simulink model "VS_1_FPNSC_Ilimit_ok"  (R2013a)
settings: Solver=ode23tb  StartTime=0.0  StopTime=.65  RelTol=1e-3
PreLoadFcn:
  | t1=1;
InitFcn:
  | t_Pref1=0.07; Pref1=10e5;
  | t_Pref2=0.3;   Pref2=3e5;
  | 
  | t_Qmax1=.12; t_Qmax2=t_Qmax1+.01;
  | t_Qref1=0.09; Qref1=7e5;
  | t_Qref2=0.5; Qref2=10e5;
  | 
  | t_Imax1=.2; Imax1=1200;
  | t_Imax2=.4; Imax2=1500;
  | 
  | t_k1=0.25; k1=.8;
  | t_k2=0.35; k2=.2;
  | t_h1=0.45; h1=.9;
  | t_h2=0.55; h2=.5;
  | 
  | Lg=90e-6;
  | l=100e-6; r=2e-3;
  | tff=10e-6;
  | w=2*pi*60;
  | z_lead =966.3602;
  | p_lead =5.6324e+03;
  | Vdc=10000;
  | Vs=690;
undefined symbols (not defined in the file): magnitude
libraries: powerlib x39, powerlib_meascontrol x17, simulink x8, simulink_extras x3
settings Model: Creator=Shahed Mortazavian  LastModifiedBy=Shahed Mortazavian
settings DataIOCC: SignalLoggingSaveFormat=ModelDataLogs
settings OptimizationCC: ExpressionDepthLimit=2147483647
settings DebuggingCC: FcnCallInpInsideContextMsg=UseLocalSettings
settings GRTTargetCC: CombineOutputUpdateFcns=off  GRTInterface=on

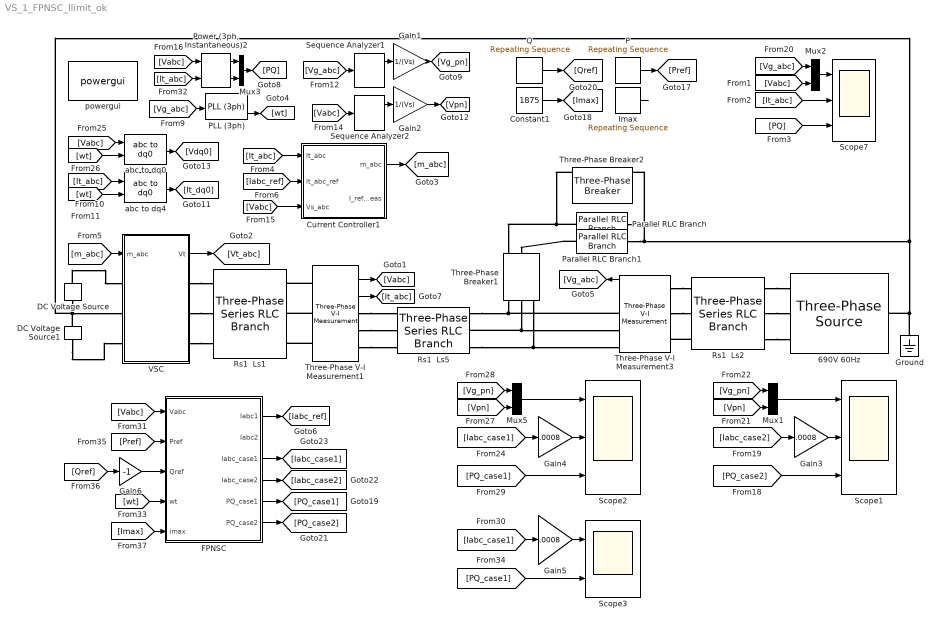
== system VS_1_FPNSC_Ilimit_ok ==
  690V 60Hz : powerlib/Electrical Sources/Three-Phase Source  Voltage=Vs*sqrt(3)/sqrt(2)  PhaseAngle=0  Frequency=60  InternalConnection=Yn  SpecifyImpedance=off  Resistance=2e-10  Inductance=1e-10  ShortCircuitLevel=100e6  BaseVoltage=25e3  XRratio=7  BusType=swing  Pref=0  Qref=0  Qmin=-inf  Qmax=inf
  Constant1 : Constant  Value=1875
  Current Controller1 : Subsystem
  DC Voltage Source : powerlib/Electrical Sources/DC Voltage Source  Amplitude=Vdc/2  Measurements=None
  DC Voltage Source1 : powerlib/Electrical Sources/DC Voltage Source  Amplitude=Vdc/2  Measurements=None
  FPNSC : Subsystem
  Gain1 : Gain  Gain=1/(Vs)
  Gain2 : Gain  Gain=1/(Vs)
  Gain3 : Gain  Gain=.0008
  Gain4 : Gain  Gain=.0008
  Gain5 : Gain  Gain=.0008
  Gain6 : Gain  Gain=-1
  Ground : powerlib/Elements/Ground  LConnTagsString=a
  Imax : simulink/Sources/Repeating Sequence  rep_seq_t=[0 t_Imax1 t_Imax1 t_Imax2 t_Imax2 10]  rep_seq_y=[1000 1000 Imax1 Imax1 Imax2 Imax2]
  Mux{1..3,5} (4 alike) : Mux  Inputs=2
  P : simulink/Sources/Repeating Sequence  rep_seq_t=[0 t_Pref1 t_Pref1 t_Pref2 t_Pref2 10]  rep_seq_y=2/3*[0 0 Pref1 Pref1 Pref2 Pref2]
  PLL (3ph) : powerlib_meascontrol/PLL/PLL (3ph)  Fmin=45  Par_Init=[0, 60]  ParK=[180, 3200, 1]  TcD=1e-4  MaxRateChangeFreq=12  FilterCutOffFreq=25  Ts=0  AGC=on
  Parallel RLC Branch : powerlib/Elements/Parallel RLC Branch  LConnTagsString=a  RConnTagsString=__new0  BranchType=R  Resistance=.8e-3  Inductance=1e-3  SetiL0=off  InitialCurrent=0  Capacitance=1e-6  Setx0=off  InitialVoltage=0  Measurements=None
  Parallel RLC Branch1 : powerlib/Elements/Parallel RLC Branch  LConnTagsString=a  RConnTagsString=__new0  BranchType=R  Resistance=.02  Inductance=1e-3  SetiL0=off  InitialCurrent=0  Capacitance=1e-6  Setx0=off  InitialVoltage=0  Measurements=None
  "Power (3ph, Instantaneous)2" : powerlib_meascontrol/Measurements/Power (3ph, Instantaneous)
  Q : simulink/Sources/Repeating Sequence  rep_seq_t=[0 t_Qref1 t_Qref1 t_Qref2 t_Qref2 10]  rep_seq_y=-2/3*[0 0 Qref1 Qref1 Qref2 Qref2]
  Rs1  Ls1 : powerlib/Elements/Three-Phase Series RLC Branch  LConnTagsString=A|B|C  RConnTagsString=A|B|C  BranchType=RL  Resistance=r  Inductance=l  Capacitance=1e-6  Measurements=None
  Rs1  Ls2 : powerlib/Elements/Three-Phase Series RLC Branch  LConnTagsString=A|B|C  RConnTagsString=A|B|C  BranchType=R  Resistance=1e-3  Inductance=l  Capacitance=1e-6  Measurements=None
  Rs1  Ls5 : powerlib/Elements/Three-Phase Series RLC Branch  LConnTagsString=A|B|C  RConnTagsString=A|B|C  BranchType=RL  Resistance=7e-3  Inductance=Lg  Capacitance=1e-6  Measurements=None
  Scope1 : Scope  NumInputPorts=3
      settings: YMin=2.77556e-17~-1~-1  YMax=1.1~1~1  SaveName=Data  Decimation=100  SampleInput=on
  Scope2 : Scope  NumInputPorts=3
      settings: YMin=2.77556e-17~-1~-500000  YMax=1.05~1~2.75e+06  SaveName=data_case1  Decimation=100  SampleInput=on
  Scope3 : Scope  NumInputPorts=2
      settings: YMin=-2~-1.5e+06  YMax=2~5.5e+06  SaveName=Data2  Decimation=100  SampleInput=on
  Scope7 : Scope  NumInputPorts=3
      settings: YMin=-1500~-1250~-1e+06  YMax=2000~1750~3e+06  SaveName=ScopeData9  Decimation=100  SampleInput=on
  Sequence Analyzer1 : powerlib_meascontrol/Measurements/Sequence Analyzer  Freq=60  n=1  seq=Positive Negative Zero  InInit=[1, 0]  Ts=0
  Sequence Analyzer2 : powerlib_meascontrol/Measurements/Sequence Analyzer  Freq=60  n=1  seq=Positive Negative Zero  InInit=[1, 0]  Ts=0
  Three-Phase V-I Measurement1 : powerlib/Measurements/Three-Phase V-I Measurement  VoltageMeasurement=phase-to-ground  SetLabelV=off  LabelV=Vabc  Vpu=off  VpuLL=off  CurrentMeasurement=yes  SetLabelI=off  LabelI=Iabc  Ipu=off  Pbase=100e6  Vbase=500e3  OutputType=Complex  PhasorSimulation=off  PSBequivalent=0
  Three-Phase V-I Measurement3 : powerlib/Measurements/Three-Phase V-I Measurement  VoltageMeasurement=phase-to-ground  SetLabelV=off  LabelV=Vabc  Vpu=off  VpuLL=off  CurrentMeasurement=yes  SetLabelI=off  LabelI=Iabc  Ipu=off  Pbase=100e6  Vbase=500e3  OutputType=Complex  PhasorSimulation=off  PSBequivalent=0
  Three-Phase Breaker1 : powerlib/Elements/Three-Phase Breaker  InitialState=open  SwitchA=on  SwitchB=on  SwitchC=on  SwitchTimes=[.2 10]  External=off  BreakerResistance=1e-40  SnubberResistance=1e6  SnubberCapacitance=inf  Measurements=None
  Three-Phase Breaker2 : powerlib/Elements/Three-Phase Breaker  InitialState=open  SwitchA=on  SwitchB=on  SwitchC=on  SwitchTimes=.4  External=off  BreakerResistance=1e-40  SnubberResistance=1e6  SnubberCapacitance=inf  Measurements=None
  VSC : Subsystem
  abc to dq0 : powerlib_meascontrol/Transformations/abc to dq0  Alignment=90 degrees behind phase A axis
  abc to dq4 : powerlib_meascontrol/Transformations/abc to dq0  Alignment=90 degrees behind phase A axis
  powergui : powerlib/powergui  Priority=2  SimulationMode=Discrete  SolverType=Tustin  SampleTime=5e-5  frequency=60  SPID=off  DisableSnubberDevices=off  DisableRonSwitches=off  DisableVfSwitches=off  SwTol=0  Interpol=off  DisplayEquations=off  frequencyindice=0  Pbase=100e6  ErrMax=1e-4  Iterations=50  UnitsV=kV  UnitsW=MW  FunctionMessages=off  echomessages=off  HookPort=off  EnableUseOfTLC=off  x0status=blocks  RestoreLinks=warning  ResistiveCurrentMeasurement=off  Frange=[0:2:500]  Ylog=off  Xlog=on  ShowGrid=off  save=off  variable=ZData  structure=Data  ZoomFFT=off  StartTime=.22  cycles=2  DisplayStyle=1  fundamental=60  FreqAxis=off  MaxFrequency=1000  frequencyindicesteady=1  RmsSteady=1  display=off  Ts=0  methode=off
  wires:
  "Power (3ph, Instantaneous)2"/1 -> Mux3/1
  "Power (3ph, Instantaneous)2"/2 -> Mux3/2
  Mux3/1 -> [PQ]
  [It_abc] -> Scope7/2
  [PQ] -> Scope7/3
  [Vg_abc] -> Sequence Analyzer1/1
  Sequence Analyzer1/1 -> Gain1/1
  Gain1/1 -> [Vg_pn]
  Three-Phase V-I Measurement1/1 -> [Vabc]
  VSC/1(Vt) -> [Vt_abc]
  [m_abc] -> VSC/1(m_abc)
  Three-Phase V-I Measurement3/1 -> [Vg_abc]
  [Vabc] -> abc to dq0/1
  [wt] -> abc to dq0/2
  abc to dq0/1 -> [Vdq0]
  [It_abc] -> abc to dq4/1
  abc to dq4/1 -> [It_dq0]
  [wt] -> abc to dq4/2
  [Vg_abc] -> PLL (3ph)/1
  [Vabc] -> "Power (3ph, Instantaneous)2"/1
  [It_abc] -> "Power (3ph, Instantaneous)2"/2
  PLL (3ph)/2 -> [wt]
  P/1 -> [Pref]
  Imax/1 -> ?
  Q/1 -> [Qref]
  Constant1/1 -> [Imax]
  [Vpn] -> Mux1/2
  [Vg_pn] -> Mux1/1
  [PQ_case2] -> Scope1/3
  Gain3/1 -> Scope1/2
  Mux1/1 -> Scope1/1
  Three-Phase V-I Measurement1/2 -> [It_abc]
  Mux2/1 -> Scope7/1
  [Vabc] -> Mux2/2
  [Vg_abc] -> Mux2/1
  [Vabc] -> Sequence Analyzer2/1
  Sequence Analyzer2/1 -> Gain2/1
  Gain2/1 -> [Vpn]
  [Iabc_case2] -> Gain3/1
  [Vpn] -> Mux5/2
  [Vg_pn] -> Mux5/1
  Mux5/1 -> Scope2/1
  Gain4/1 -> Scope2/2
  [Iabc_case1] -> Gain4/1
  [PQ_case1] -> Scope2/3
  Gain5/1 -> Scope3/1
  [Iabc_case1] -> Gain5/1
  [PQ_case1] -> Scope3/2
  [wt] -> FPNSC/4(wt)
  [Vabc] -> FPNSC/1(Vabc)
  [Pref] -> FPNSC/2(Pref)
  [Qref] -> Gain6/1
  [Imax] -> FPNSC/5(imax)
  FPNSC/3(Iabc_case1) -> [Iabc_case1]
  FPNSC/4(Iabc_case2) -> [Iabc_case2]
  FPNSC/5(PQ_case1) -> [PQ_case1]
  FPNSC/6(PQ_case2) -> [PQ_case2]
  [It_abc] -> Current Controller1/1(It_abc)
  [Vabc] -> Current Controller1/3(Vs_abc)
  Current Controller1/1(m_abc) -> [m_abc]
  FPNSC/1(Iabc1) -> [Iabc_ref]
  [Iabc_ref] -> Current Controller1/2(It_abc_ref)
  Gain6/1 -> FPNSC/3(Qref)
  connections:
  Three-Phase V-I Measurement1/LConn1 -- Rs1  Ls1/RConn1
  Three-Phase V-I Measurement1/LConn2 -- Rs1  Ls1/RConn2
  Three-Phase V-I Measurement1/LConn3 -- Rs1  Ls1/RConn3
  Rs1  Ls5/RConn1 -- Three-Phase V-I Measurement3/RConn1 -- Three-Phase Breaker1/LConn1
  Three-Phase Breaker2/LConn1 -- Parallel RLC Branch/LConn1 -- Three-Phase Breaker1/RConn1
  VSC/RConn1 -- Rs1  Ls1/LConn1
  VSC/RConn2 -- Rs1  Ls1/LConn2
  VSC/RConn3 -- Rs1  Ls1/LConn3
  DC Voltage Source/RConn1 -- VSC/LConn1
  DC Voltage Source1/LConn1 -- VSC/LConn3
  Three-Phase Breaker1/LConn2 -- Rs1  Ls5/RConn2 -- Three-Phase V-I Measurement3/RConn2
  Rs1  Ls5/RConn3 -- Three-Phase Breaker1/LConn3 -- Three-Phase V-I Measurement3/RConn3
  Three-Phase V-I Measurement3/LConn1 -- Rs1  Ls2/LConn1
  Three-Phase V-I Measurement3/LConn2 -- Rs1  Ls2/LConn2
  Rs1  Ls2/LConn3 -- Three-Phase V-I Measurement3/LConn3
  Rs1  Ls2/RConn1 -- 690V 60Hz/RConn1
  Rs1  Ls2/RConn2 -- 690V 60Hz/RConn2
  Rs1  Ls2/RConn3 -- 690V 60Hz/RConn3
  Parallel RLC Branch1/LConn1 -- Three-Phase Breaker1/RConn2
  Three-Phase V-I Measurement1/RConn1 -- Rs1  Ls5/LConn1
  Three-Phase V-I Measurement1/RConn2 -- Rs1  Ls5/LConn2
  Three-Phase V-I Measurement1/RConn3 -- Rs1  Ls5/LConn3
  DC Voltage Source/LConn1 -- DC Voltage Source1/RConn1 -- Parallel RLC Branch1/RConn1 -- Three-Phase Breaker2/RConn1 -- Parallel RLC Branch/RConn1 -- Ground/LConn1 -- 690V 60Hz/LConn1 -- VSC/LConn2

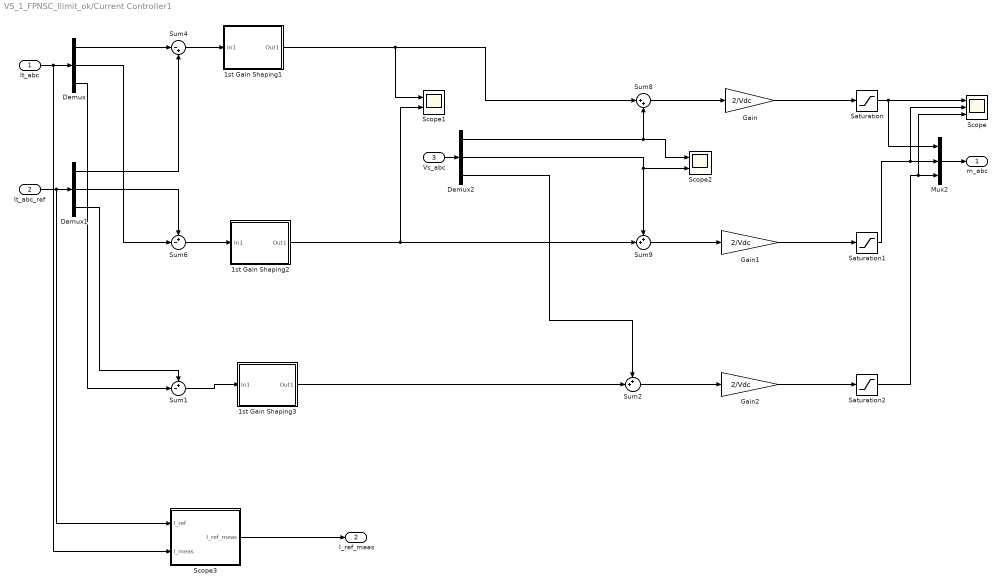
== system VS_1_FPNSC_Ilimit_ok/Current Controller1 ==
  It_abc : Inport
  It_abc_ref : Inport  Port=2
  Vs_abc : Inport  Port=3
  1st Gain Shaping1 : Subsystem
  1st Gain Shaping2 : Subsystem
  1st Gain Shaping3 : Subsystem
  Demux : Demux  Outputs=3
  Demux1 : Demux  Outputs=3
  Demux2 : Demux  Outputs=3
  Gain : Gain  Gain=2/Vdc
  Gain1 : Gain  Gain=2/Vdc
  Gain2 : Gain  Gain=2/Vdc
  Mux2 : Mux  Inputs=3
  Saturation : Saturate  UpperLimit=1  LowerLimit=-1
  Saturation1 : Saturate  UpperLimit=1  LowerLimit=-1
  Saturation2 : Saturate  UpperLimit=1  LowerLimit=-1
  Scope : Scope  NumInputPorts=3
      settings: YMin=-0.7~-1~-0.75  YMax=0.8~0.75~1  SaveName=ScopeData4  Decimation=3
  Scope1 : Scope  NumInputPorts=2
      settings: YMin=-1600~-200  YMax=400~600  SaveName=ScopeData3  Decimation=3
  Scope2 : Scope  NumInputPorts=2
      settings: YMin=-400~-450  YMax=400~400  SaveName=ScopeData5  Decimation=3
  Scope3 : Subsystem
  Sum1 : Sum  Inputs=+-|
  Sum2 : Sum  Inputs=++|
  Sum4 : Sum  Inputs=|-+
  Sum6 : Sum  Inputs=+-|
  Sum8 : Sum  Inputs=|++
  Sum9 : Sum  Inputs=++|
  m_abc : Outport
  I_ref_meas : Outport  Port=2
  wires:
  Demux2/1 -> Scope2/1, Sum8/2
  Demux2/2 -> Scope2/2, Sum9/1
  Sum6/1 -> 1st Gain Shaping2/1(In1)
  It_abc/1 -> Scope3/2(I_meas), Demux/1
  It_abc_ref/1 -> Scope3/1(I_ref), Demux1/1
  Vs_abc/1 -> Demux2/1
  Sum8/1 -> Gain/1
  Sum9/1 -> Gain1/1
  Mux2/1 -> m_abc/1
  Gain/1 -> Saturation/1
  Gain1/1 -> Saturation1/1
  Saturation2/1 -> Scope/3, Mux2/3
  Saturation/1 -> Scope/1, Mux2/1
  Saturation1/1 -> Mux2/2, Scope/2
  Demux1/1 -> Sum4/2
  Demux/1 -> Sum4/1
  Sum4/1 -> 1st Gain Shaping1/1(In1)
  Demux1/2 -> Sum6/1
  Demux/2 -> Sum6/2
  Demux1/3 -> Sum1/1
  Demux/3 -> Sum1/2
  Sum1/1 -> 1st Gain Shaping3/1(In1)
  Gain2/1 -> Saturation2/1
  Sum2/1 -> Gain2/1
  Demux2/3 -> Sum2/1
  1st Gain Shaping2/1(Out1) -> Scope1/2, Sum9/2
  1st Gain Shaping3/1(Out1) -> Sum2/2
  1st Gain Shaping1/1(Out1) -> Scope1/1, Sum8/1
  Scope3/1(I_ref_meas) -> I_ref_meas/1

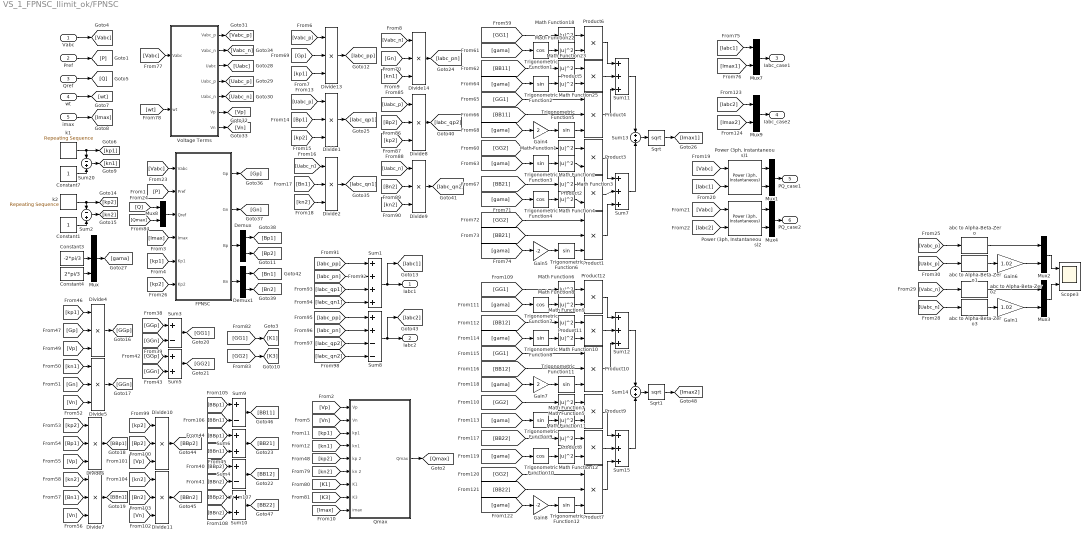
== system VS_1_FPNSC_Ilimit_ok/FPNSC ==
  Vabc : Inport
  Pref : Inport  Port=2
  Qref : Inport  Port=3
  wt : Inport  Port=4
  imax : Inport  Port=5
  Constant1 : Constant
  Constant3 : Constant  Value=-2*pi/3
  Constant4 : Constant  Value=2*pi/3
  Constant7 : Constant
  Demux : Demux  Outputs=2
  Demux1 : Demux  Outputs=2
  Divide{1..2,4..11,13..14} (12 alike) : Product  Inputs=***
  FPNSC : Subsystem
  Gain1 : Gain  Gain=1.02
  Gain4 : Gain  Gain=2
  Gain5 : Gain  Gain=-2
  Gain6 : Gain  Gain=1.02
  Gain7 : Gain  Gain=2
  Gain8 : Gain  Gain=-2
  Math Function{1..12,18,22..23,25} (16 alike) : Math  Operator=magnitude^2  SaturateOnIntegerOverflow=on
  Mux : Mux  Inputs=3
  Mux{1..4,7..9} (7 alike) : Mux  Inputs=2
  "Power (3ph, Instantaneous)1" : powerlib_meascontrol/Measurements/Power (3ph, Instantaneous)
  "Power (3ph, Instantaneous)2" : powerlib_meascontrol/Measurements/Power (3ph, Instantaneous)
  Product{1,4,7,10} (4 alike) : Product  Inputs=3
  Product{2..3,5..6,8..9,11..12} (8 alike) : Product
  Qmax : Subsystem
  Scope3 : Scope  NumInputPorts=2
      settings: YMin=-800~-70  YMax=800~70  SaveName=ScopeData11
  Sqrt : Sqrt  SaturateOnIntegerOverflow=on
  Sqrt1 : Sqrt  SaturateOnIntegerOverflow=on
  Sum1 : Sum  Inputs=++++
  Sum{5..6,10,13..14} (5 alike) : Sum
  Sum{7,11..12,15} (4 alike) : Sum  Inputs=+++
  Sum2 : Sum  Inputs=-+
  Sum20 : Sum  Inputs=-+
  Sum3 : Sum  Inputs=+-
  Sum4 : Sum  Inputs=+-
  Sum8 : Sum  Inputs=++--
  Sum9 : Sum  Inputs=+-
  Trigonometric Function{1,4,7,10} (4 alike) : Trigonometry  Operator=cos
  Trigonometric Function{2..3,5..6,8..9,11..12} (8 alike) : Trigonometry
  Voltage Terms : Subsystem
  abc to Alpha-Beta-Zero{,1..3} (4 alike) : powerlib_meascontrol/Transformations/abc to Alpha-Beta-Zero
  k1 : simulink/Sources/Repeating Sequence  rep_seq_t=[0 t_k1 t_k1 t_k2 t_k2 10]  rep_seq_y=[1 1 k1 k1 k2 k2]
  k2 : simulink/Sources/Repeating Sequence  rep_seq_t=[0 t_h1 t_h1 t_h2 t_h2 10]  rep_seq_y=[1 1 h1 h1 h2 h2]
  Iabc1 : Outport
  Iabc2 : Outport  Port=2
  Iabc_case1 : Outport  Port=3
  Iabc_case2 : Outport  Port=4
  PQ_case1 : Outport  Port=5
  PQ_case2 : Outport  Port=6
  wires:
  Divide13/1 -> [Iabc_pp]
  [kp1] -> FPNSC/5(Kp1)
  [Imax] -> FPNSC/4(Imax)
  [P] -> FPNSC/2(Pref)
  [Vabc] -> FPNSC/1(Vabc)
  Mux1/1 -> PQ_case1/1
  "Power (3ph, Instantaneous)1"/2 -> Mux1/2
  "Power (3ph, Instantaneous)1"/1 -> Mux1/1
  [Iabc1] -> "Power (3ph, Instantaneous)1"/2
  [Vabc] -> "Power (3ph, Instantaneous)1"/1
  Sum1/1 -> Iabc1/1, [Iabc1]
  [kn2] -> Divide2/3
  [Bn1] -> Divide2/2
  [Uabc_n] -> Divide2/1
  [kp2] -> Divide1/3
  [Uabc_p] -> Divide1/1
  [kn1] -> Divide14/3
  [Vabc_n] -> Divide14/1
  [kp1] -> Divide13/3
  Sum20/1 -> [kn1]
  k1/1 -> [kp1], Sum20/1
  [Vabc_p] -> Divide13/1
  imax/1 -> [Imax]
  wt/1 -> [wt]
  Qref/1 -> [Q]
  Pref/1 -> [P]
  Vabc/1 -> [Vabc]
  FPNSC/4(Bn) -> Demux1/1
  FPNSC/2(Gn) -> [Gn]
  Constant7/1 -> Sum20/2
  [Gp] -> Divide13/2
  [Gn] -> Divide14/2
  [Vabc_p] -> abc to Alpha-Beta-Zero/1
  [Uabc_p] -> abc to Alpha-Beta-Zero1/1
  [Vabc_n] -> abc to Alpha-Beta-Zero2/1
  [Uabc_n] -> abc to Alpha-Beta-Zero3/1
  abc to Alpha-Beta-Zero/1 -> Mux2/1
  abc to Alpha-Beta-Zero1/1 -> Gain6/1
  abc to Alpha-Beta-Zero2/1 -> Mux3/1
  abc to Alpha-Beta-Zero3/1 -> Gain1/1
  Mux2/1 -> Scope3/1
  Mux3/1 -> Scope3/2
  Gain6/1 -> Mux2/2
  Gain1/1 -> Mux3/2
  Sum2/1 -> [kn2]
  k2/1 -> Sum2/1, [kp2]
  Constant1/1 -> Sum2/2
  [kp2] -> FPNSC/6(Kp2)
  [GGp] -> Sum3/1
  [GGn] -> Sum3/2
  Sum3/1 -> [GG1]
  [BBp2] -> Sum4/1
  [BBn2] -> Sum4/2
  Sum4/1 -> [BB12]
  [GGp] -> Sum5/1
  [GGn] -> Sum5/2
  Sum5/1 -> [GG2]
  [BBp1] -> Sum6/1
  [BBn1] -> Sum6/2
  Sum6/1 -> [BB21]
  [kp1] -> Divide4/1
  [Gp] -> Divide4/2
  [Vp] -> Divide4/3
  Divide4/1 -> [GGp]
  [kn1] -> Divide5/1
  [Gn] -> Divide5/2
  [Vn] -> Divide5/3
  Divide5/1 -> [GGn]
  Divide6/1 -> [BBp1]
  Divide7/1 -> [BBn1]
  [kp2] -> Divide6/1
  [Bp1] -> Divide6/2
  [Vp] -> Divide6/3
  [Vn] -> Divide7/3
  [Bn1] -> Divide7/2
  [kn2] -> Divide7/1
  [GG1] -> Math Function18/1
  [gama] -> Trigonometric Function1/1
  Trigonometric Function1/1 -> Math Function22/1
  Math Function22/1 -> Product6/2
  Math Function18/1 -> Product6/1
  Math Function23/1 -> Product5/1
  Math Function25/1 -> Product5/2
  [BB11] -> Math Function23/1
  [gama] -> Trigonometric Function2/1
  Trigonometric Function2/1 -> Math Function25/1
  [GG1] -> Product4/1
  [BB11] -> Product4/2
  [gama] -> Gain4/1
  Product6/1 -> Sum11/1
  Product5/1 -> Sum11/2
  Product4/1 -> Sum11/3
  Sum11/1 -> Sum13/1
  Sum7/1 -> Sum13/2
  Sum13/1 -> Sqrt/1
  Gain4/1 -> Trigonometric Function5/1
  Trigonometric Function5/1 -> Product4/3
  [GG2] -> Math Function1/1
  [gama] -> Trigonometric Function3/1
  Trigonometric Function3/1 -> Math Function2/1
  Math Function2/1 -> Product3/2
  Math Function1/1 -> Product3/1
  Math Function3/1 -> Product2/1
  Math Function4/1 -> Product2/2
  [BB21] -> Math Function3/1
  [gama] -> Trigonometric Function4/1
  Trigonometric Function4/1 -> Math Function4/1
  [GG2] -> Product1/1
  [BB21] -> Product1/2
  [gama] -> Gain5/1
  Product3/1 -> Sum7/1
  Product2/1 -> Sum7/2
  Product1/1 -> Sum7/3
  Gain5/1 -> Trigonometric Function6/1
  Trigonometric Function6/1 -> Product1/3
  [Iabc1] -> Mux7/1
  Sqrt/1 -> [Imax1]
  [Imax1] -> Mux7/2
  Mux7/1 -> Iabc_case1/1
  Constant3/1 -> Mux/2
  Constant4/1 -> Mux/3
  Mux/1 -> [gama]
  [wt] -> Voltage Terms/2(wt)
  [Vabc] -> Voltage Terms/1(Vabc)
  Voltage Terms/1(Vabc_p) -> [Vabc_p]
  Voltage Terms/2(Vabc_n) -> [Vabc_n]
  Voltage Terms/3(Uabc) -> [Uabc]
  Voltage Terms/4(Uabc_p) -> [Uabc_p]
  Voltage Terms/5(Uabc_n) -> [Uabc_n]
  Voltage Terms/6(Vp) -> [Vp]
  Voltage Terms/7(Vn) -> [Vn]
  [Vn] -> Qmax/2(Vn)
  [kp1] -> Qmax/3(kp1)
  [Vp] -> Qmax/1(Vp)
  [Imax] -> Qmax/9(imax)
  Qmax/1(Qmax) -> [Qmax]
  [kn1] -> Qmax/4(kn1)
  [kp2] -> Qmax/5(kp 2)
  [kn2] -> Qmax/6(kn 2)
  [K1] -> Qmax/7(K1)
  [K3] -> Qmax/8(K3)
  [GG1] -> [K1]
  [GG2] -> [K3]
  [Q] -> Mux8/1
  [Qmax] -> Mux8/2
  Mux8/1 -> FPNSC/3(Qref)
  FPNSC/1(Gp) -> [Gp]
  FPNSC/3(Bp) -> Demux/1
  Demux/1 -> [Bp1]
  Demux/2 -> [Bp2]
  Divide14/1 -> [Iabc_pn]
  Divide1/1 -> [Iabc_qp1]
  [Bp1] -> Divide1/2
  Divide2/1 -> [Iabc_qn1]
  [kn2] -> Divide9/3
  [Bn2] -> Divide9/2
  [Uabc_n] -> Divide9/1
  [kp2] -> Divide8/3
  [Uabc_p] -> Divide8/1
  Divide8/1 -> [Iabc_qp2]
  [Bp2] -> Divide8/2
  Divide9/1 -> [Iabc_qn2]
  Demux1/1 -> [Bn1]
  Demux1/2 -> [Bn2]
  [Iabc_pp] -> Sum1/1
  [Iabc_pn] -> Sum1/2
  [Iabc_qp1] -> Sum1/3
  [Iabc_qn1] -> Sum1/4
  Sum8/1 -> Iabc2/1, [Iabc2]
  [Iabc_pp] -> Sum8/1
  [Iabc_pn] -> Sum8/2
  [Iabc_qp2] -> Sum8/3
  [Iabc_qn2] -> Sum8/4
  Divide10/1 -> [BBp2]
  Divide11/1 -> [BBn2]
  [kp2] -> Divide10/1
  [Bp2] -> Divide10/2
  [Vp] -> Divide10/3
  [Vn] -> Divide11/3
  [Bn2] -> Divide11/2
  [kn2] -> Divide11/1
  [BBp1] -> Sum9/1
  [BBn1] -> Sum9/2
  Sum9/1 -> [BB11]
  [BBp2] -> Sum10/1
  [BBn2] -> Sum10/2
  Sum10/1 -> [BB22]
  [GG1] -> Math Function6/1
  [gama] -> Trigonometric Function7/1
  Trigonometric Function7/1 -> Math Function8/1
  Math Function8/1 -> Product12/2
  Math Function6/1 -> Product12/1
  Math Function9/1 -> Product11/1
  Math Function10/1 -> Product11/2
  [BB12] -> Math Function9/1
  [gama] -> Trigonometric Function8/1
  Trigonometric Function8/1 -> Math Function10/1
  [GG1] -> Product10/1
  [BB12] -> Product10/2
  [gama] -> Gain7/1
  Product12/1 -> Sum12/1
  Product11/1 -> Sum12/2
  Product10/1 -> Sum12/3
  Sum12/1 -> Sum14/1
  Sum15/1 -> Sum14/2
  Sum14/1 -> Sqrt1/1
  Gain7/1 -> Trigonometric Function11/1
  Trigonometric Function11/1 -> Product10/3
  [GG2] -> Math Function5/1
  [gama] -> Trigonometric Function9/1
  Trigonometric Function9/1 -> Math Function7/1
  Math Function7/1 -> Product9/2
  Math Function5/1 -> Product9/1
  Math Function11/1 -> Product8/1
  Math Function12/1 -> Product8/2
  [BB22] -> Math Function11/1
  [gama] -> Trigonometric Function10/1
  Trigonometric Function10/1 -> Math Function12/1
  [GG2] -> Product7/1
  [BB22] -> Product7/2
  [gama] -> Gain8/1
  Product9/1 -> Sum15/1
  Product8/1 -> Sum15/2
  Product7/1 -> Sum15/3
  Gain8/1 -> Trigonometric Function12/1
  Trigonometric Function12/1 -> Product7/3
  Sqrt1/1 -> [Imax2]
  [Iabc2] -> Mux9/1
  [Imax2] -> Mux9/2
  Mux9/1 -> Iabc_case2/1
  Mux4/1 -> PQ_case2/1
  "Power (3ph, Instantaneous)2"/2 -> Mux4/2
  "Power (3ph, Instantaneous)2"/1 -> Mux4/1
  [Iabc2] -> "Power (3ph, Instantaneous)2"/2
  [Vabc] -> "Power (3ph, Instantaneous)2"/1

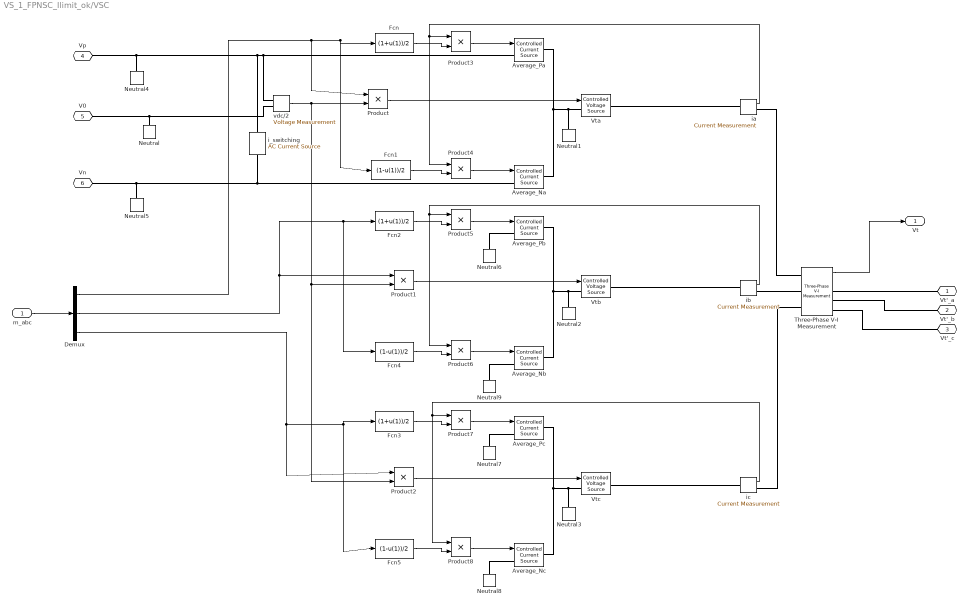
== system VS_1_FPNSC_Ilimit_ok/VSC ==
  m_abc : Inport
  Average_Na : powerlib/Electrical Sources/Controlled Current Source  Initialize=on  Source_Type=AC  Amplitude=0  Phase=0  Frequency=0  Measurements=None
  Average_Nb : powerlib/Electrical Sources/Controlled Current Source  Initialize=on  Source_Type=AC  Amplitude=0  Phase=0  Frequency=0  Measurements=None
  Average_Nc : powerlib/Electrical Sources/Controlled Current Source  Initialize=on  Source_Type=AC  Amplitude=0  Phase=0  Frequency=0  Measurements=None
  Average_Pa : powerlib/Electrical Sources/Controlled Current Source  Initialize=on  Source_Type=AC  Amplitude=0  Phase=0  Frequency=0  Measurements=None
  Average_Pb : powerlib/Electrical Sources/Controlled Current Source  Initialize=on  Source_Type=AC  Amplitude=0  Phase=0  Frequency=0  Measurements=None
  Average_Pc : powerlib/Electrical Sources/Controlled Current Source  Initialize=on  Source_Type=AC  Amplitude=0  Phase=0  Frequency=0  Measurements=None
  Demux : Demux  Outputs=3
  Fcn : Fcn  Expr=(1+u(1))/2
  Fcn1 : Fcn  Expr=(1-u(1))/2
  Fcn2 : Fcn  Expr=(1+u(1))/2
  Fcn3 : Fcn  Expr=(1+u(1))/2
  Fcn4 : Fcn  Expr=(1-u(1))/2
  Fcn5 : Fcn  Expr=(1-u(1))/2
  Neutral{,1..3} (4 alike) : powerlib/Elements/Neutral  LConnTagsString=a  NodeNumber=10
  Neutral4 : powerlib/Elements/Neutral  LConnTagsString=a  NodeNumber=11
  Neutral5 : powerlib/Elements/Neutral  LConnTagsString=a  NodeNumber=12
  Neutral6 : powerlib/Elements/Neutral  LConnTagsString=a  NodeNumber=11
  Neutral7 : powerlib/Elements/Neutral  LConnTagsString=a  NodeNumber=11
  Neutral8 : powerlib/Elements/Neutral  LConnTagsString=a  NodeNumber=12
  Neutral9 : powerlib/Elements/Neutral  LConnTagsString=a  NodeNumber=12
  Product{,1..8} (9 alike) : Product  RndMeth=Zero
  Three-Phase V-I Measurement : powerlib/Measurements/Three-Phase V-I Measurement  VoltageMeasurement=phase-to-ground  SetLabelV=off  LabelV=Vabc  Vpu=off  VpuLL=off  CurrentMeasurement=yes  SetLabelI=off  LabelI=Iabc  Ipu=off  Pbase=100e6  Vbase=500e3  OutputType=Complex  PhasorSimulation=off  PSBequivalent=0
  Vta : powerlib/Electrical Sources/Controlled Voltage Source  Initialize=on  Source_Type=AC  Amplitude=0  Phase=0  Frequency=0  Measurements=None
  Vtb : powerlib/Electrical Sources/Controlled Voltage Source  Initialize=on  Source_Type=AC  Amplitude=0  Phase=0  Frequency=0  Measurements=None
  Vtc : powerlib/Electrical Sources/Controlled Voltage Source  Initialize=on  Source_Type=AC  Amplitude=0  Phase=0  Frequency=0  Measurements=None
  i_switching : powerlib/Electrical Sources/AC Current Source  Amplitude=1  Phase=0  Frequency=0  SampleTime=0  Measurements=None
  ia : powerlib/Measurements/Current Measurement  PhasorSimulation=off  OutputType=Complex  PSBequivalent=0
  ib : powerlib/Measurements/Current Measurement  PhasorSimulation=off  OutputType=Complex  PSBequivalent=0
  ic : powerlib/Measurements/Current Measurement  PhasorSimulation=off  OutputType=Complex  PSBequivalent=0
  vdc/2 : powerlib/Measurements/Voltage Measurement  PhasorSimulation=off  OutputType=Complex  PSBequivalent=0
  Vt'_a : PMIOPort  Port=1  Side=Right
  Vt'_b : PMIOPort  Port=2  Side=Right
  Vt'_c : PMIOPort  Port=3  Side=Right
  Vp : PMIOPort  Port=4  Side=Left
  V0 : PMIOPort  Port=5  Side=Left
  Vn : PMIOPort  Port=6  Side=Left
  Vt : Outport
  wires:
  Fcn1/1 -> Product4/2
  Fcn2/1 -> Product5/2
  Fcn4/1 -> Product6/2
  Fcn3/1 -> Product7/2
  Fcn5/1 -> Product8/2
  Demux/1 -> Fcn/1, Fcn1/1, Product/1
  Demux/2 -> Fcn2/1, Fcn4/1, Product1/1
  Demux/3 -> Fcn3/1, Fcn5/1, Product2/1
  vdc/2/1 -> Product/2, Product1/2, Product2/2
  Product/1 -> Vta/1
  Product1/1 -> Vtb/1
  Product2/1 -> Vtc/1
  Product3/1 -> Average_Pa/1
  Fcn/1 -> Product3/2
  Product4/1 -> Average_Na/1
  Product5/1 -> Average_Pb/1
  Product7/1 -> Average_Pc/1
  Product8/1 -> Average_Nc/1
  ia/1 -> Product3/1, Product4/1
  ib/1 -> Product5/1, Product6/1
  ic/1 -> Product7/1, Product8/1
  Product6/1 -> Average_Nb/1
  m_abc/1 -> Demux/1
  Three-Phase V-I Measurement/1 -> Vt/1
  connections:
  Vn/RConn1 -- i_switching/RConn1 -- Average_Na/LConn1 -- Neutral5/LConn1
  Vp/RConn1 -- vdc/2/LConn1 -- Average_Pa/LConn1 -- i_switching/LConn1 -- Neutral4/LConn1
  Vta/RConn1 -- ia/LConn1
  Vtb/RConn1 -- ib/LConn1
  Vtc/RConn1 -- ic/LConn1
  Average_Pb/RConn1 -- Average_Nb/RConn1 -- Vtb/LConn1 -- Neutral2/LConn1
  Three-Phase V-I Measurement/LConn1 -- ia/RConn1
  Three-Phase V-I Measurement/LConn2 -- ib/RConn1
  Three-Phase V-I Measurement/LConn3 -- ic/RConn1
  Average_Pa/RConn1 -- Average_Na/RConn1 -- Vta/LConn1 -- Neutral1/LConn1
  Average_Pc/RConn1 -- Average_Nc/RConn1 -- Vtc/LConn1 -- Neutral3/LConn1
  V0/RConn1 -- vdc/2/LConn2 -- Neutral/LConn1
  Neutral6/LConn1 -- Average_Pb/LConn1
  Neutral7/LConn1 -- Average_Pc/LConn1
  Neutral8/LConn1 -- Average_Nc/LConn1
  Neutral9/LConn1 -- Average_Nb/LConn1
  Vt'_a/RConn1 -- Three-Phase V-I Measurement/RConn1
  Three-Phase V-I Measurement/RConn2 -- Vt'_b/RConn1
  Three-Phase V-I Measurement/RConn3 -- Vt'_c/RConn1

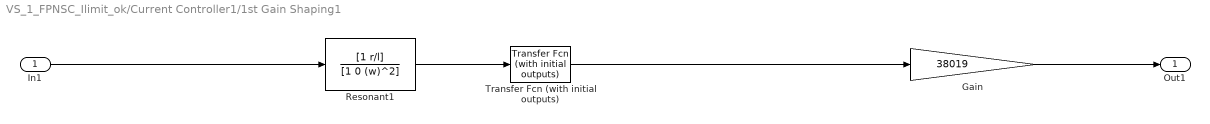
== system VS_1_FPNSC_Ilimit_ok/Current Controller1/1st Gain Shaping1 ==
  In1 : Inport
  Gain : Gain  Gain=38019
  Resonant1 : TransferFcn  Numerator=[1 r/l]  Denominator=[1 0 (w)^2]
  Transfer Fcn (with initial outputs) : simulink_extras/Additional Linear/Transfer Fcn (with initial outputs)  N=[1 5205]  D=[1 30340]  Y0=0  U0=0
  Out1 : Outport
  wires:
  Resonant1/1 -> Transfer Fcn (with initial outputs)/1
  In1/1 -> Resonant1/1
  Gain/1 -> Out1/1
  Transfer Fcn (with initial outputs)/1 -> Gain/1

== system VS_1_FPNSC_Ilimit_ok/Current Controller1/1st Gain Shaping2 ==
  In1 : Inport
  Gain : Gain  Gain=38019
  Resonant1 : TransferFcn  Numerator=[1 r/l]  Denominator=[1 0 (w)^2]
  Transfer Fcn (with initial outputs) : simulink_extras/Additional Linear/Transfer Fcn (with initial outputs)  N=[1 5205]  D=[1 30340]  Y0=0  U0=0
  Out1 : Outport
  wires:
  Transfer Fcn (with initial outputs)/1 -> Gain/1
  Gain/1 -> Out1/1
  In1/1 -> Resonant1/1
  Resonant1/1 -> Transfer Fcn (with initial outputs)/1

== system VS_1_FPNSC_Ilimit_ok/Current Controller1/1st Gain Shaping3 ==
  In1 : Inport
  Gain : Gain  Gain=38019
  Resonant1 : TransferFcn  Numerator=[1 r/l]  Denominator=[1 0 (w)^2]
  Transfer Fcn (with initial outputs) : simulink_extras/Additional Linear/Transfer Fcn (with initial outputs)  N=[1 5205]  D=[1 30340]  Y0=0  U0=0
  Out1 : Outport
  wires:
  Resonant1/1 -> Transfer Fcn (with initial outputs)/1
  In1/1 -> Resonant1/1
  Gain/1 -> Out1/1
  Transfer Fcn (with initial outputs)/1 -> Gain/1

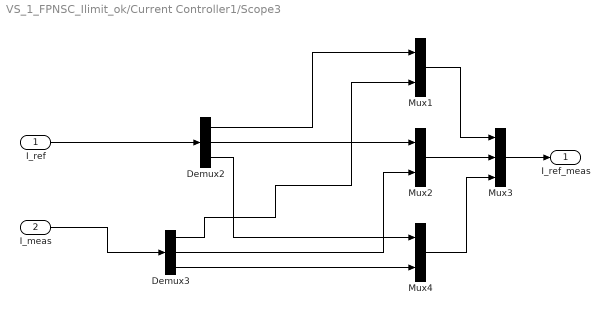
== system VS_1_FPNSC_Ilimit_ok/Current Controller1/Scope3 ==
  I_ref : Inport
  I_meas : Inport  Port=2
  Demux2 : Demux  Outputs=3
  Demux3 : Demux  Outputs=3
  Mux1 : Mux  Inputs=2
  Mux2 : Mux  Inputs=2
  Mux3 : Mux  Inputs=3
  Mux4 : Mux  Inputs=2
  I_ref_meas : Outport
  wires:
  I_meas/1 -> Demux3/1
  I_ref/1 -> Demux2/1
  Demux2/1 -> Mux1/1
  Demux3/1 -> Mux1/2
  Mux1/1 -> Mux3/1
  Demux2/2 -> Mux2/1
  Demux3/2 -> Mux2/2
  Mux2/1 -> Mux3/2
  Demux2/3 -> Mux4/1
  Demux3/3 -> Mux4/2
  Mux4/1 -> Mux3/3
  Mux3/1 -> I_ref_meas/1

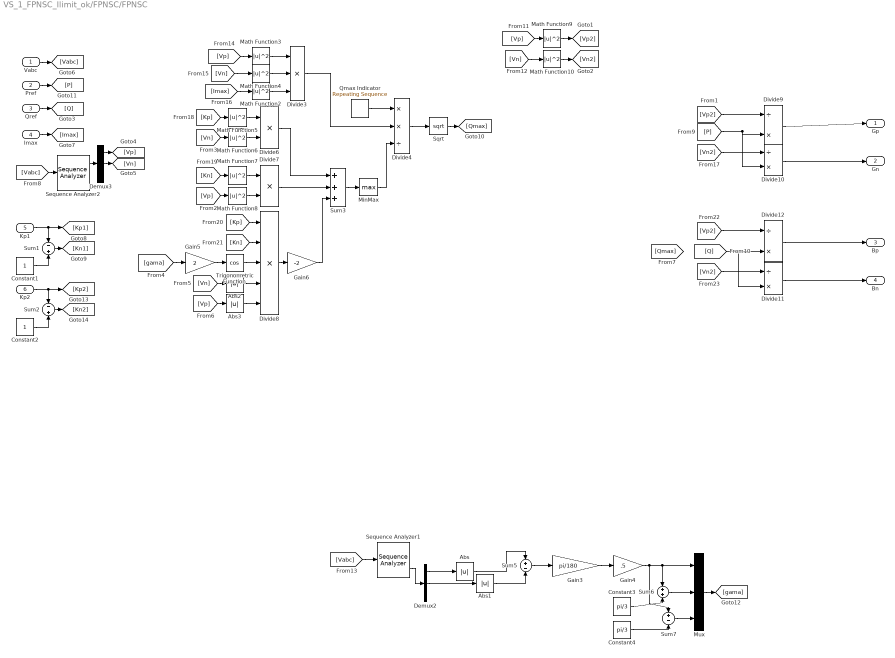
== system VS_1_FPNSC_Ilimit_ok/FPNSC/FPNSC ==
  Vabc : Inport
  Pref : Inport  Port=2
  Qref : Inport  Port=3
  Imax : Inport  Port=4
  Kp1 : Inport  Port=5
  Kp2 : Inport  Port=6
  Abs{,1..3} (4 alike) : Abs
  Constant1 : Constant
  Constant2 : Constant
  Constant3 : Constant  Value=pi/3
  Constant4 : Constant  Value=pi/3
  Demux2 : Demux  Outputs=3
  Demux3 : Demux  Outputs=3
  Divide{9..12} (4 alike) : Product  Inputs=/*
  Divide3 : Product  Inputs=***
  Divide4 : Product  Inputs=**/
  Divide6 : Product  Inputs=**
  Divide7 : Product  Inputs=**
  Divide8 : Product  Inputs=*****
  Gain3 : Gain  Gain=pi/180
  Gain4 : Gain  Gain=.5
  Gain5 : Gain  Gain=2
  Gain6 : Gain  Gain=-2
  Math Function{2..10} (9 alike) : Math  Operator=magnitude^2  SaturateOnIntegerOverflow=on
  MinMax : MinMax  Function=max
  Mux : Mux  Inputs=3
  Qmax Indicator : simulink/Sources/Repeating Sequence  rep_seq_t=[0 t_Qmax1 t_Qmax2 10]  rep_seq_y=[0 0 1 1]
  Sequence Analyzer1 : powerlib_meascontrol/Measurements/Sequence Analyzer  Freq=60  n=1  seq=Positive Negative Zero  InInit=[1, 0]  Ts=0
  Sequence Analyzer2 : powerlib_meascontrol/Measurements/Sequence Analyzer  Freq=60  n=1  seq=Positive Negative Zero  InInit=[1, 0]  Ts=0
  Sqrt : Sqrt  SaturateOnIntegerOverflow=on
  Sum1 : Sum  Inputs=-+
  Sum2 : Sum  Inputs=-+
  Sum3 : Sum  Inputs=+++
  Sum5 : Sum  Inputs=+-
  Sum6 : Sum
  Sum7 : Sum  Inputs=+-
  Trigonometric Function : Trigonometry  Operator=cos
  Gp : Outport
  Gn : Outport  Port=2
  Bp : Outport  Port=3
  Bn : Outport  Port=4
  wires:
  Qref/1 -> [Q]
  Sum6/1 -> Mux/2
  Sum7/1 -> Mux/3
  Mux/1 -> [gama]
  Pref/1 -> [P]
  [Q] -> Divide12/2, Divide11/2
  Sqrt/1 -> [Qmax]
  [Kn] -> Math Function7/1
  Sum1/1 -> [Kn1]
  Constant1/1 -> Sum1/2
  Kp1/1 -> Sum1/1, [Kp1]
  [Imax] -> Math Function2/1
  [Vn] -> Math Function4/1
  [Vp] -> Math Function3/1
  [Vabc] -> Sequence Analyzer1/1
  Qmax Indicator/1 -> Divide4/1
  Math Function8/1 -> Divide7/2
  Divide4/1 -> Sqrt/1
  MinMax/1 -> Divide4/3
  [Kn] -> Divide8/2
  [Kp] -> Divide8/1
  Gain6/1 -> Sum3/3
  Divide8/1 -> Gain6/1
  Abs3/1 -> Divide8/5
  Abs2/1 -> Divide8/4
  [Vp] -> Abs3/1
  [Vn] -> Abs2/1
  Gain5/1 -> Trigonometric Function/1
  Trigonometric Function/1 -> Divide8/3
  [gama] -> Gain5/1
  Constant4/1 -> Sum7/2
  Constant3/1 -> Sum6/2
  Gain4/1 -> Sum7/1, Mux/1, Sum6/1
  Gain3/1 -> Gain4/1
  Sum5/1 -> Gain3/1
  Abs1/1 -> Sum5/2
  Abs/1 -> Sum5/1
  Demux2/2 -> Abs1/1
  Demux2/1 -> Abs/1
  Sequence Analyzer1/2 -> Demux2/1
  Divide7/1 -> Sum3/2
  [Vp] -> Math Function8/1
  Math Function7/1 -> Divide7/1
  Divide6/1 -> Sum3/1
  Math Function6/1 -> Divide6/2
  [Vn] -> Math Function6/1
  Math Function5/1 -> Divide6/1
  [Kp] -> Math Function5/1
  Sum3/1 -> MinMax/1
  Divide3/1 -> Divide4/2
  Math Function4/1 -> Divide3/2
  Math Function3/1 -> Divide3/1
  Math Function2/1 -> Divide3/3
  Imax/1 -> [Imax]
  Vabc/1 -> [Vabc]
  [P] -> Divide10/2, Divide9/2
  Divide9/1 -> Gp/1
  Divide10/1 -> Gn/1
  Divide12/1 -> Bp/1
  Divide11/1 -> Bn/1
  [Vabc] -> Sequence Analyzer2/1
  Sequence Analyzer2/1 -> Demux3/1
  Demux3/1 -> [Vp]
  Demux3/2 -> [Vn]
  [Vp] -> Math Function9/1
  [Vn] -> Math Function10/1
  Math Function9/1 -> [Vp2]
  Math Function10/1 -> [Vn2]
  [Vp2] -> Divide9/1
  [Vn2] -> Divide10/1
  [Vp2] -> Divide12/1
  [Vn2] -> Divide11/1
  Sum2/1 -> [Kn2]
  Constant2/1 -> Sum2/2
  Kp2/1 -> [Kp2], Sum2/1

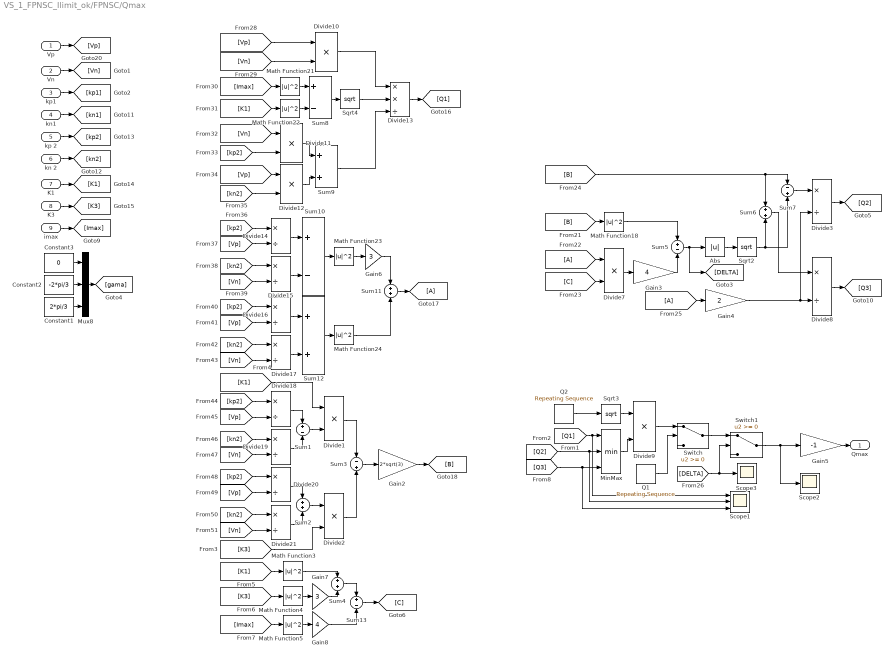
== system VS_1_FPNSC_Ilimit_ok/FPNSC/Qmax ==
  Vp : Inport
  Vn : Inport  Port=2
  kp1 : Inport  Port=3
  kn1 : Inport  Port=4
  kp 2 : Inport  Port=5
  kn 2 : Inport  Port=6
  K1 : Inport  Port=7
  K3 : Inport  Port=8
  imax : Inport  Port=9
  Abs : Abs
  Constant1 : Constant  Value=2*pi/3
  Constant2 : Constant  Value=-2*pi/3
  Constant3 : Constant  Value=0
  Divide{1..2,7,9..12} (7 alike) : Product  Inputs=**
  Divide13 : Product  Inputs=**/
  Divide{3,8,14..21} (10 alike) : Product  Inputs=*/
  Gain2 : Gain  Gain=2*sqrt(3)
  Gain3 : Gain  Gain=4
  Gain4 : Gain  Gain=2
  Gain5 : Gain  Gain=-1
  Gain6 : Gain  Gain=3
  Gain7 : Gain  Gain=3
  Gain8 : Gain  Gain=4
  Math Function{3..5,18,21..24} (8 alike) : Math  Operator=magnitude^2  SaturateOnIntegerOverflow=on
  MinMax : MinMax  Inputs=3
  Mux8 : Mux  Inputs=3
  Q1 : simulink/Sources/Repeating Sequence  rep_seq_t=[0 t_Qmax1 t_Qmax1 10]  rep_seq_y=[-1 -1 1 1]
  Q2 : simulink/Sources/Repeating Sequence  rep_seq_t=[0 t_Qmax1 t_Qmax2 10]  rep_seq_y=[0 0 1 1]
  Scope1 : Scope  NumInputPorts=3
      settings: YMin=0~-100000~0  YMax=1.3e+06~1.3e+06~1.7e+06
  Scope2 : Scope
      settings: YMin=0  YMax=1.2e+06  SaveName=ScopeData10
  Scope3 : Scope
      settings: YMin=0  YMax=1.2e+06
  Sqrt2 : Sqrt  SaturateOnIntegerOverflow=on
  Sqrt3 : Sqrt  SaturateOnIntegerOverflow=on
  Sqrt4 : Sqrt  SaturateOnIntegerOverflow=on
  Sum{1,5,8,10,13} (5 alike) : Sum  Inputs=+-
  Sum{2,4,6,9,11..12} (6 alike) : Sum
  Sum3 : Sum  Inputs=-+
  Sum7 : Sum  Inputs=-+
  Switch : Switch
  Switch1 : Switch
  Qmax : Outport
  wires:
  kp1/1 -> [kp1]
  Vn/1 -> [Vn]
  Vp/1 -> [Vp]
  imax/1 -> [Imax]
  [B] -> Math Function18/1
  Math Function18/1 -> Sum5/1
  [A] -> Divide7/1
  [C] -> Divide7/2
  Divide7/1 -> Gain3/1
  Gain3/1 -> Sum5/2
  Abs/1 -> Sqrt2/1
  Sqrt2/1 -> Sum7/2, Sum6/2
  [B] -> Sum7/1, Sum6/1
  Sum6/1 -> Divide8/1
  [A] -> Gain4/1
  Gain4/1 -> Divide8/2, Divide3/2
  Constant1/1 -> Mux8/3
  Constant3/1 -> Mux8/1
  Constant2/1 -> Mux8/2
  Mux8/1 -> [gama]
  MinMax/1 -> Divide9/2
  Switch/1 -> Switch1/1
  Q1/1 -> Switch/2
  Switch1/1 -> Scope2/1, Gain5/1
  Sum5/1 -> Abs/1, [DELTA]
  Gain5/1 -> Qmax/1
  Q2/1 -> Sqrt3/1
  Divide9/1 -> Switch/1
  Sqrt3/1 -> Divide9/1
  Divide8/1 -> [Q3]
  [DELTA] -> Scope3/1, Switch1/2
  kn1/1 -> [kn1]
  kp 2/1 -> [kp2]
  kn 2/1 -> [kn2]
  K1/1 -> [K1]
  K3/1 -> [K3]
  [Vn] -> Divide10/2
  [Vp] -> Divide10/1
  [Imax] -> Math Function21/1
  Math Function21/1 -> Sum8/1
  [K1] -> Math Function22/1
  Math Function22/1 -> Sum8/2
  [Vn] -> Divide11/1
  [kp2] -> Divide11/2
  [Vp] -> Divide12/1
  [kn2] -> Divide12/2
  Divide11/1 -> Sum9/1
  Divide12/1 -> Sum9/2
  Divide10/1 -> Divide13/1
  Sum8/1 -> Sqrt4/1
  Sum9/1 -> Divide13/3
  Divide13/1 -> [Q1]
  Sqrt4/1 -> Divide13/2
  [kp2] -> Divide14/1
  [Vp] -> Divide14/2
  [kn2] -> Divide15/1
  [Vn] -> Divide15/2
  Divide14/1 -> Sum10/1
  Divide15/1 -> Sum10/2
  Sum10/1 -> Math Function23/1
  Math Function23/1 -> Gain6/1
  Gain6/1 -> Sum11/1
  [kp2] -> Divide16/1
  [Vp] -> Divide16/2
  [kn2] -> Divide17/1
  [Vn] -> Divide17/2
  Divide16/1 -> Sum12/1
  Divide17/1 -> Sum12/2
  Sum12/1 -> Math Function24/1
  Math Function24/1 -> Sum11/2
  Sum11/1 -> [A]
  [kp2] -> Divide18/1
  [Vp] -> Divide18/2
  [kn2] -> Divide19/1
  [Vn] -> Divide19/2
  Divide18/1 -> Sum1/1
  Divide19/1 -> Sum1/2
  [kp2] -> Divide20/1
  [Vp] -> Divide20/2
  [kn2] -> Divide21/1
  [Vn] -> Divide21/2
  Divide20/1 -> Sum2/1
  Divide21/1 -> Sum2/2
  Sum3/1 -> Gain2/1
  Gain2/1 -> [B]
  Sum1/1 -> Divide1/2
  [K1] -> Divide1/1
  Sum2/1 -> Divide2/1
  [K3] -> Divide2/2
  Divide1/1 -> Sum3/1
  Divide2/1 -> Sum3/2
  [K1] -> Math Function3/1
  Math Function3/1 -> Sum4/1
  [K3] -> Math Function4/1
  Math Function4/1 -> Gain7/1
  Gain7/1 -> Sum4/2
  Sum4/1 -> Sum13/1
  Gain8/1 -> Sum13/2
  Math Function5/1 -> Gain8/1
  [Imax] -> Math Function5/1
  Sum13/1 -> [C]
  Sum7/1 -> Divide3/1
  Divide3/1 -> [Q2]
  [Q1] -> Scope1/1, MinMax/1
  [Q2] -> Scope1/2, MinMax/2
  [Q3] -> Scope1/3, MinMax/3

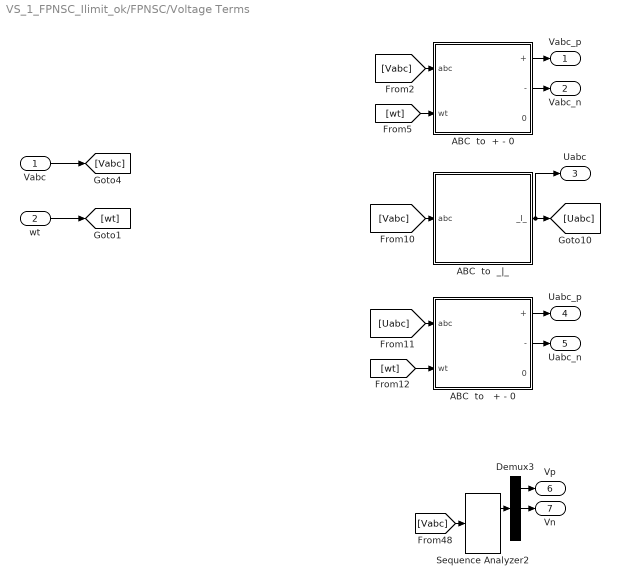
== system VS_1_FPNSC_Ilimit_ok/FPNSC/Voltage Terms ==
  Vabc : Inport
  wt : Inport  Port=2
  ABC  to   + - 0 : Subsystem
  ABC  to  + - 0 : Subsystem
  ABC  to  _|_ : Subsystem
  Demux3 : Demux  Outputs=3
  Sequence Analyzer2 : powerlib_meascontrol/Measurements/Sequence Analyzer  Freq=60  n=1  seq=Positive Negative Zero  InInit=[1, 0]  Ts=0
  Vabc_p : Outport
  Vabc_n : Outport  Port=2
  Uabc : Outport  Port=3
  Uabc_p : Outport  Port=4
  Uabc_n : Outport  Port=5
  Vp : Outport  Port=6
  Vn : Outport  Port=7
  wires:
  wt/1 -> [wt]
  ABC  to   + - 0/2(-) -> Uabc_n/1
  ABC  to   + - 0/1(+) -> Uabc_p/1
  [wt] -> ABC  to   + - 0/2(wt)
  [Uabc] -> ABC  to   + - 0/1(abc)
  ABC  to  _|_/1(_I_) -> Uabc/1, [Uabc]
  [Vabc] -> ABC  to  _|_/1(abc)
  [wt] -> ABC  to  + - 0/2(wt)
  [Vabc] -> ABC  to  + - 0/1(abc)
  ABC  to  + - 0/1(+) -> Vabc_p/1
  ABC  to  + - 0/2(-) -> Vabc_n/1
  [Vabc] -> Sequence Analyzer2/1
  Sequence Analyzer2/1 -> Demux3/1
  Demux3/1 -> Vp/1
  Demux3/2 -> Vn/1
  Vabc/1 -> [Vabc]

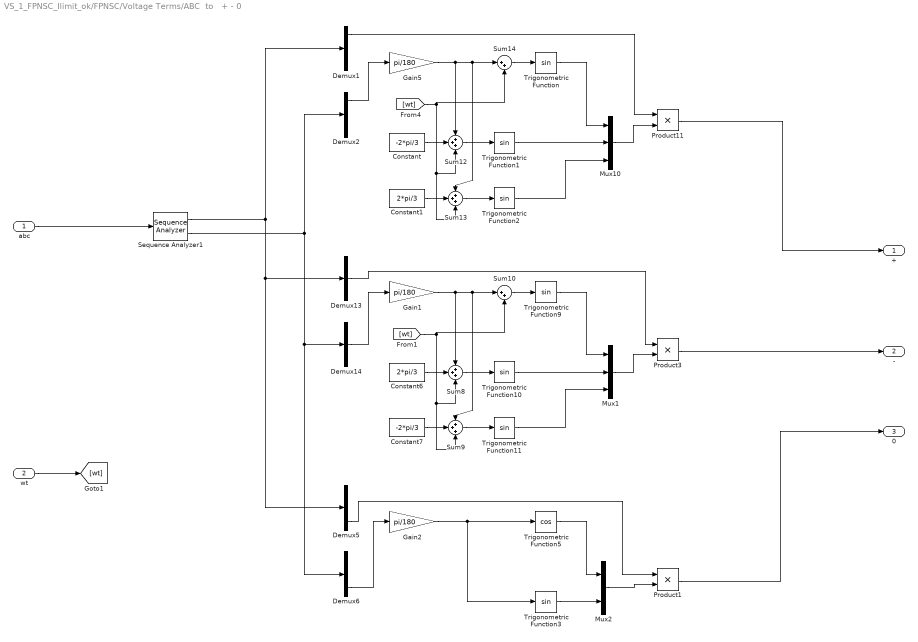
== system VS_1_FPNSC_Ilimit_ok/FPNSC/Voltage Terms/ABC  to   + - 0 ==
  abc : Inport
  wt : Inport  Port=2
  Constant : Constant  Value=-2*pi/3
  Constant1 : Constant  Value=2*pi/3
  Constant6 : Constant  Value=2*pi/3
  Constant7 : Constant  Value=-2*pi/3
  Demux{1..2,5..6,13..14} (6 alike) : Demux  Outputs=3
  Gain1 : Gain  Gain=pi/180
  Gain2 : Gain  Gain=pi/180
  Gain5 : Gain  Gain=pi/180
  Mux1 : Mux  Inputs=3
  Mux10 : Mux  Inputs=3
  Mux2 : Mux  Inputs=2
  Product1 : Product
  Product11 : Product
  Product3 : Product
  Sequence Analyzer1 : powerlib_meascontrol/Measurements/Sequence Analyzer  Freq=60  n=1  seq=Positive Negative Zero  InInit=[1, 0]  Ts=0
  Sum10 : Sum  Inputs=|++
  Sum{8..9,12..13} (4 alike) : Sum  Inputs=+++
  Sum14 : Sum  Inputs=|++
  Trigonometric Function{,1..3,9..11} (7 alike) : Trigonometry
  Trigonometric Function5 : Trigonometry  Operator=cos
  + : Outport
  - : Outport  Port=2
  0 : Outport  Port=3
  wires:
  Trigonometric Function/1 -> Mux10/1
  Constant/1 -> Sum12/2
  Sum12/1 -> Trigonometric Function1/1
  Trigonometric Function1/1 -> Mux10/2
  Constant1/1 -> Sum13/2
  Sum13/1 -> Trigonometric Function2/1
  Trigonometric Function2/1 -> Mux10/3
  Mux10/1 -> Product11/2
  Demux1/1 -> Product11/1
  Demux2/1 -> Gain5/1
  Sum14/1 -> Trigonometric Function/1
  Gain5/1 -> Sum12/1, Sum13/1, Sum14/1
  wt/1 -> [wt]
  abc/1 -> Sequence Analyzer1/1
  [wt] -> Sum13/3, Sum12/3, Sum14/2
  Trigonometric Function9/1 -> Mux1/1
  Constant6/1 -> Sum8/2
  Sum8/1 -> Trigonometric Function10/1
  Trigonometric Function10/1 -> Mux1/2
  Constant7/1 -> Sum9/2
  Sum9/1 -> Trigonometric Function11/1
  Trigonometric Function11/1 -> Mux1/3
  Mux1/1 -> Product3/2
  Demux13/2 -> Product3/1
  Demux14/2 -> Gain1/1
  Sum10/1 -> Trigonometric Function9/1
  Gain1/1 -> Sum10/1, Sum9/1, Sum8/1
  [wt] -> Sum10/2, Sum8/3, Sum9/3
  Sequence Analyzer1/1 -> Demux1/1, Demux5/1, Demux13/1
  Sequence Analyzer1/2 -> Demux2/1, Demux6/1, Demux14/1
  Trigonometric Function5/1 -> Mux2/1
  Trigonometric Function3/1 -> Mux2/2
  Mux2/1 -> Product1/2
  Demux5/3 -> Product1/1
  Demux6/3 -> Gain2/1
  Gain2/1 -> Trigonometric Function5/1, Trigonometric Function3/1
  Product11/1 -> +/1
  Product3/1 -> -/1
  Product1/1 -> 0/1

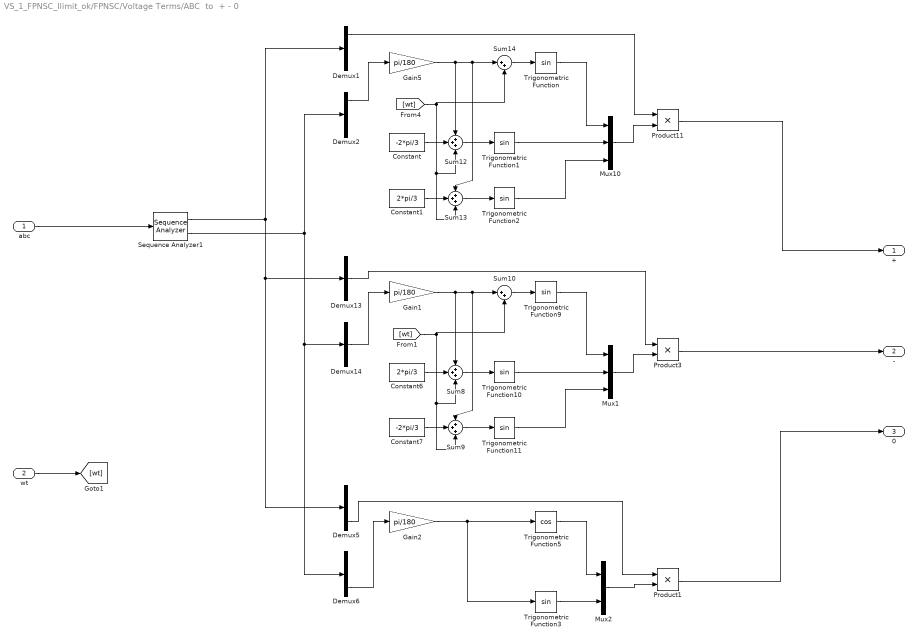
== system VS_1_FPNSC_Ilimit_ok/FPNSC/Voltage Terms/ABC  to  + - 0 ==
  abc : Inport
  wt : Inport  Port=2
  Constant : Constant  Value=-2*pi/3
  Constant1 : Constant  Value=2*pi/3
  Constant6 : Constant  Value=2*pi/3
  Constant7 : Constant  Value=-2*pi/3
  Demux{1..2,5..6,13..14} (6 alike) : Demux  Outputs=3
  Gain1 : Gain  Gain=pi/180
  Gain2 : Gain  Gain=pi/180
  Gain5 : Gain  Gain=pi/180
  Mux1 : Mux  Inputs=3
  Mux10 : Mux  Inputs=3
  Mux2 : Mux  Inputs=2
  Product1 : Product
  Product11 : Product
  Product3 : Product
  Sequence Analyzer1 : powerlib_meascontrol/Measurements/Sequence Analyzer  Freq=60  n=1  seq=Positive Negative Zero  InInit=[1, 0]  Ts=0
  Sum10 : Sum  Inputs=|++
  Sum{8..9,12..13} (4 alike) : Sum  Inputs=+++
  Sum14 : Sum  Inputs=|++
  Trigonometric Function{,1..3,9..11} (7 alike) : Trigonometry
  Trigonometric Function5 : Trigonometry  Operator=cos
  + : Outport
  - : Outport  Port=2
  0 : Outport  Port=3
  wires:
  Trigonometric Function/1 -> Mux10/1
  Constant/1 -> Sum12/2
  Sum12/1 -> Trigonometric Function1/1
  Trigonometric Function1/1 -> Mux10/2
  Constant1/1 -> Sum13/2
  Sum13/1 -> Trigonometric Function2/1
  Trigonometric Function2/1 -> Mux10/3
  Mux10/1 -> Product11/2
  Demux1/1 -> Product11/1
  Demux2/1 -> Gain5/1
  Sum14/1 -> Trigonometric Function/1
  Gain5/1 -> Sum12/1, Sum13/1, Sum14/1
  wt/1 -> [wt]
  abc/1 -> Sequence Analyzer1/1
  [wt] -> Sum13/3, Sum12/3, Sum14/2
  Trigonometric Function9/1 -> Mux1/1
  Constant6/1 -> Sum8/2
  Sum8/1 -> Trigonometric Function10/1
  Trigonometric Function10/1 -> Mux1/2
  Constant7/1 -> Sum9/2
  Sum9/1 -> Trigonometric Function11/1
  Trigonometric Function11/1 -> Mux1/3
  Mux1/1 -> Product3/2
  Demux13/2 -> Product3/1
  Demux14/2 -> Gain1/1
  Sum10/1 -> Trigonometric Function9/1
  Gain1/1 -> Sum10/1, Sum9/1, Sum8/1
  [wt] -> Sum10/2, Sum8/3, Sum9/3
  Sequence Analyzer1/1 -> Demux1/1, Demux5/1, Demux13/1
  Sequence Analyzer1/2 -> Demux2/1, Demux6/1, Demux14/1
  Trigonometric Function5/1 -> Mux2/1
  Trigonometric Function3/1 -> Mux2/2
  Mux2/1 -> Product1/2
  Demux5/3 -> Product1/1
  Demux6/3 -> Gain2/1
  Gain2/1 -> Trigonometric Function5/1, Trigonometric Function3/1
  Product11/1 -> +/1
  Product3/1 -> -/1
  Product1/1 -> 0/1

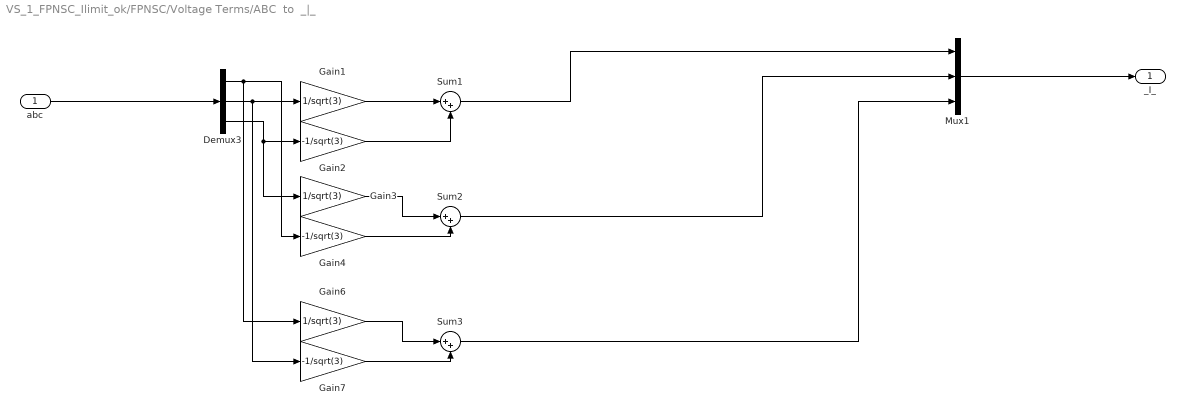
== system VS_1_FPNSC_Ilimit_ok/FPNSC/Voltage Terms/ABC  to  _|_ ==
  abc : Inport
  Demux3 : Demux  Outputs=3
  Gain1 : Gain  Gain=1/sqrt(3)
  Gain2 : Gain  Gain=-1/sqrt(3)
  Gain3 : Gain  Gain=1/sqrt(3)
  Gain4 : Gain  Gain=-1/sqrt(3)
  Gain6 : Gain  Gain=1/sqrt(3)
  Gain7 : Gain  Gain=-1/sqrt(3)
  Mux1 : Mux  Inputs=3
  Sum1 : Sum  Inputs=|++
  Sum2 : Sum  Inputs=|++
  Sum3 : Sum  Inputs=|++
  _I_ : Outport
  wires:
  Mux1/1 -> _I_/1
  abc/1 -> Demux3/1
  Demux3/2 -> Gain7/1, Gain1/1
  Demux3/3 -> Gain3/1, Gain2/1
  Sum1/1 -> Mux1/1
  Gain1/1 -> Sum1/1
  Gain2/1 -> Sum1/2
  Gain3/1 -> Sum2/1
  Gain4/1 -> Sum2/2
  Demux3/1 -> Gain6/1, Gain4/1
  Sum2/1 -> Mux1/2
  Gain6/1 -> Sum3/1
  Gain7/1 -> Sum3/2
  Sum3/1 -> Mux1/3
